simulink model "singlePhaseInverterOpenLoop"  (R2023a)
settings: Solver=VariableStepAuto  StartTime=0.0  StopTime=.2  FixedStep=1e-3  MaxStep=1e-5  RelTol=1e-3
libraries: spsIGBTDiodeLib x16, spsDCVoltageSourceLib x8, spsTHDLib x8, spsCurrentMeasurementLib x6, spsGroundLib x4, spsSeriesRLCBranchLib x4, spsVoltageMeasurementLib x4, spspowerguiLib x3, simulink x3, spsMeanLib x1, spsTriangleGeneratorLib x1
settings Model: Creator=User  LastModifiedBy=User
settings SolverCC: AlgebraicLoopSolver=TrustRegion
settings DebuggingCC: UnconnectedInputMsg=warning  UnconnectedOutputMsg=warning  UnconnectedLineMsg=warning
settings ModelReferenceCC: EnableRefExpFcnMdlSchedulingChecks=on
settings RTWCC: DLArmComputeVersion=19.05

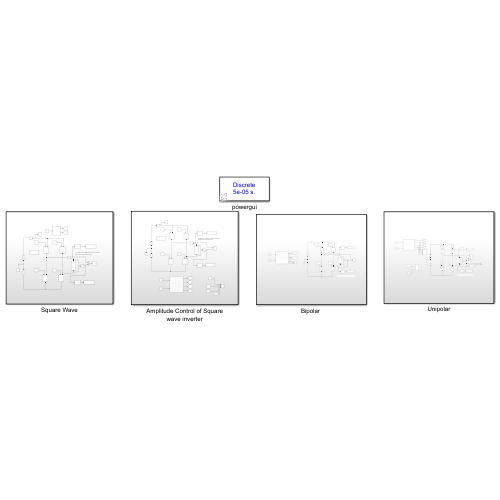
[thumbnail: Simulink's stored preview of the top-level diagram]
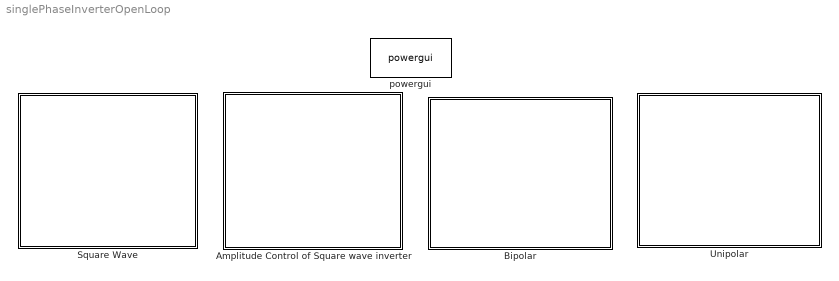
== system singlePhaseInverterOpenLoop ==
  Amplitude Control of Square wave inverter : Subsystem
  "Bipolar " : Subsystem
  Square Wave : Subsystem
  Unipolar : Subsystem
  powergui : spspowerguiLib/powergui  Priority=1  SimulationMode=Discrete  SampleTime=50e-6  frequency=60  Iterations=50  frequencyindice=0  Pbase=100e6  ErrMax=1e-4  UnitsV=kV  UnitsW=MW  buscounter=0  FunctionMessages=off  echomessages=off  EnableUseOfTLC=off  CurrentSourceSwitches=off  DisableSnubberDevices=on  DisableRonSwitches=on  DisableVfSwitches=on  DisplayEquations=off  AutomaticDiscreteSolvers=off  SolverType=Tustin/Backward Euler (TBE)  Interpol=off  ExternalGateDelay=off  methode=off  Ts=100  x0status=blocks  SPID=on  SwTol=0  HookPort=off  NonlinearTolerance=1e-4  nMaxIteration=100  ContinueOnMaxIteration=off  RestoreLinks=warning  ResistiveCurrentMeasurement=off  Frange=[0:2:500]  Ylog=off  Xlog=on  ShowGrid=off  save=off  variable=ZData  structure=0  ZoomFFT=off  StartTime=0.0  cycles=1  DisplayStyle=1  fundamental=60  FreqAxis=off  MaxFrequency=1000  frequencyindicesteady=1  RmsSteady=1  display=off

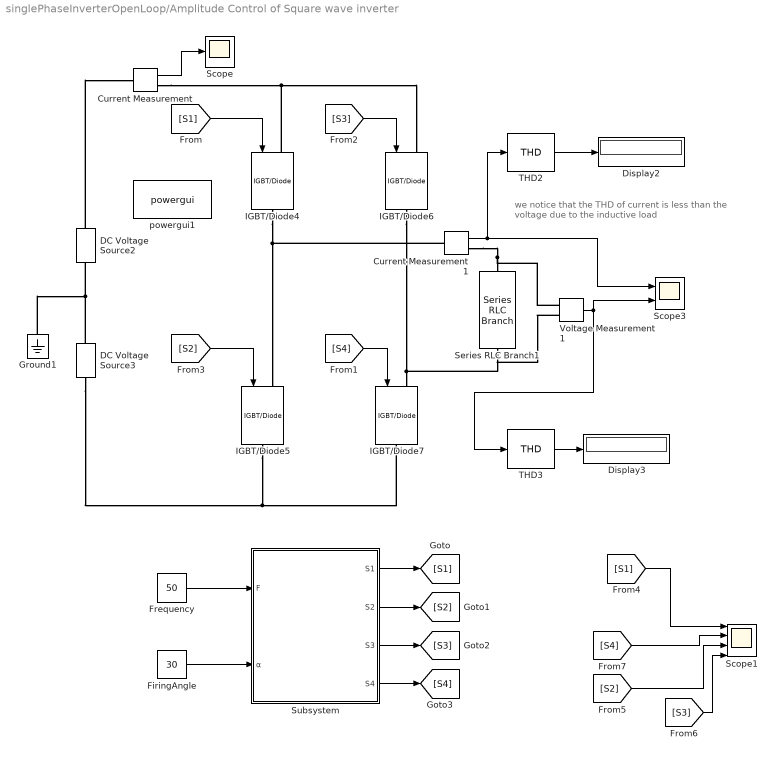
== system singlePhaseInverterOpenLoop/Amplitude Control of Square wave inverter ==
  note: we notice that the THD of current is less than the voltage due to the inductive load
  Current Measurement : spsCurrentMeasurementLib/Current Measurement  PhasorSimulation=off  OutputType=Complex  PSBequivalent=0
  Current Measurement1 : spsCurrentMeasurementLib/Current Measurement  PhasorSimulation=off  OutputType=Complex  PSBequivalent=0
  DC Voltage Source2 : spsDCVoltageSourceLib/DC Voltage Source  Amplitude=100  Measurements=None
  DC Voltage Source3 : spsDCVoltageSourceLib/DC Voltage Source  Amplitude=100  Measurements=None
  Display2 : Display
  Display3 : Display
  FiringAngle : Constant  Value=30
  Frequency : Constant  Value=50
  Ground1 : spsGroundLib/Ground  LConnTagsString=a
  IGBT/Diode{4..7} (4 alike) : spsIGBTDiodeLib/IGBT//Diode  Ron=1e-3  Rs=1e5  Cs=inf  Measurements=off
  Scope : Scope
  Scope1 : Scope  NumInputPorts=4
  Scope3 : Scope  NumInputPorts=2
  Series RLC Branch1 : spsSeriesRLCBranchLib/Series RLC Branch  LConnTagsString=__new0  RConnTagsString=__new0  BranchType=RL  Resistance=1  Inductance=1e-3  SetiL0=off  InitialCurrent=0  Capacitance=1e-6  Setx0=off  InitialVoltage=0  Measurements=None
  Subsystem : Subsystem
  THD2 : spsTHDLib/THD  Freq=60  Ts=0
  THD3 : spsTHDLib/THD  Freq=60  Ts=0
  Voltage Measurement1 : spsVoltageMeasurementLib/Voltage Measurement  PhasorSimulation=off  OutputType=Complex  PSBequivalent=0
  powergui1 : spspowerguiLib/powergui  Priority=1  SimulationMode=Continuous  SampleTime=50e-6  frequency=60  Iterations=50  frequencyindice=0  Pbase=100e6  ErrMax=1e-4  UnitsV=kV  UnitsW=MW  buscounter=0  FunctionMessages=off  echomessages=off  EnableUseOfTLC=off  CurrentSourceSwitches=off  DisableSnubberDevices=on  DisableRonSwitches=on  DisableVfSwitches=on  DisplayEquations=off  AutomaticDiscreteSolvers=off  SolverType=Tustin/Backward Euler (TBE)  Interpol=off  ExternalGateDelay=off  methode=off  Ts=100  x0status=blocks  SPID=on  SwTol=0  HookPort=off  NonlinearTolerance=1e-4  nMaxIteration=100  ContinueOnMaxIteration=off  RestoreLinks=warning  ResistiveCurrentMeasurement=off  Frange=[0:2:500]  Ylog=off  Xlog=on  ShowGrid=off  save=off  variable=ZData  structure=0  ZoomFFT=off  StartTime=0.0  cycles=1  DisplayStyle=1  fundamental=60  FreqAxis=off  MaxFrequency=1000  frequencyindicesteady=1  RmsSteady=1  display=off
  wires:
  Current Measurement/1 -> Scope/1
  [S1] -> IGBT/Diode4/1
  Voltage Measurement1/1 -> Scope3/2, THD3/1
  THD2/1 -> Display2/1
  [S2] -> IGBT/Diode5/1
  [S3] -> IGBT/Diode6/1
  THD3/1 -> Display3/1
  [S4] -> IGBT/Diode7/1
  Current Measurement1/1 -> Scope3/1, THD2/1
  Frequency/1 -> Subsystem/1(F)
  FiringAngle/1 -> Subsystem/2(α)
  Subsystem/1(S1) -> [S1]
  Subsystem/2(S2) -> [S2]
  Subsystem/3(S3) -> [S3]
  Subsystem/4(S4) -> [S4]
  [S1] -> Scope1/1
  [S2] -> Scope1/3
  [S3] -> Scope1/4
  [S4] -> Scope1/2
  connections:
  DC Voltage Source2/RConn1 -- Current Measurement/LConn1
  Voltage Measurement1/LConn1 -- Current Measurement1/RConn1 -- Series RLC Branch1/LConn1
  Ground1/LConn1 -- DC Voltage Source3/RConn1 -- DC Voltage Source2/LConn1
  IGBT/Diode6/RConn1 -- Series RLC Branch1/RConn1 -- Voltage Measurement1/LConn2 -- IGBT/Diode7/LConn1
  Current Measurement1/LConn1 -- IGBT/Diode4/RConn1 -- IGBT/Diode5/LConn1
  IGBT/Diode4/LConn1 -- Current Measurement/RConn1 -- IGBT/Diode6/LConn1
  DC Voltage Source3/LConn1 -- IGBT/Diode7/RConn1 -- IGBT/Diode5/RConn1

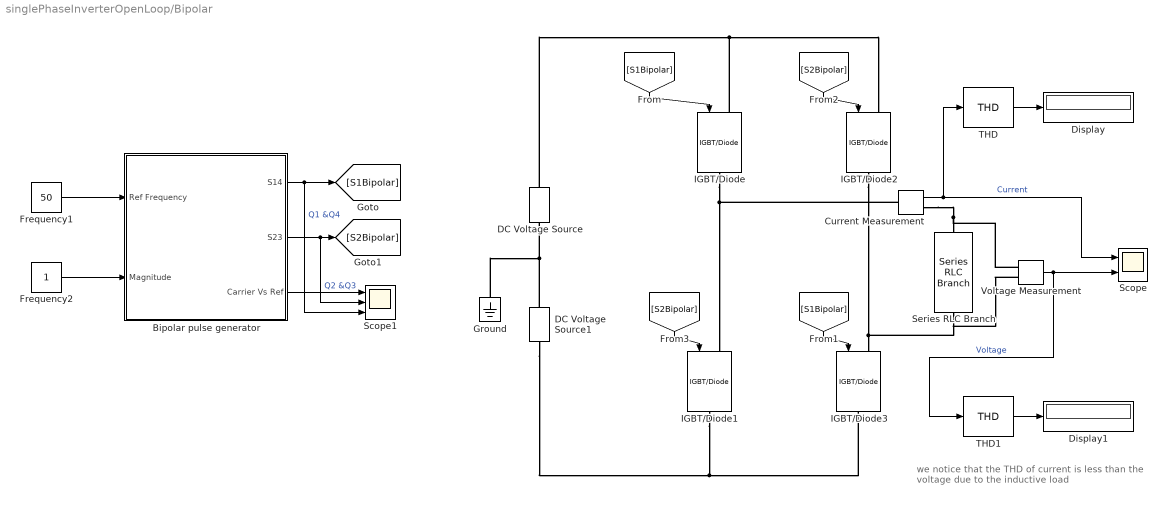
== system singlePhaseInverterOpenLoop/Bipolar  ==
  note: we notice that the THD of current is less than the voltage due to the inductive load
  Bipolar pulse generator : Subsystem
  Current Measurement : spsCurrentMeasurementLib/Current Measurement  PhasorSimulation=off  OutputType=Complex  PSBequivalent=0
  DC Voltage Source : spsDCVoltageSourceLib/DC Voltage Source  Amplitude=100  Measurements=None
  DC Voltage Source1 : spsDCVoltageSourceLib/DC Voltage Source  Amplitude=100  Measurements=None
  Display : Display
  Display1 : Display
  Frequency1 : Constant  Value=50
  Frequency2 : Constant
  Ground : spsGroundLib/Ground  LConnTagsString=a
  IGBT/Diode{,1..3} (4 alike) : spsIGBTDiodeLib/IGBT//Diode  Ron=1e-3  Rs=1e5  Cs=inf  Measurements=off
  Scope : Scope  NumInputPorts=2
  Scope1 : Scope  NumInputPorts=3
  Series RLC Branch : spsSeriesRLCBranchLib/Series RLC Branch  LConnTagsString=__new0  RConnTagsString=__new0  BranchType=RL  Resistance=1  Inductance=50e-3  SetiL0=off  InitialCurrent=0  Capacitance=1e-6  Setx0=off  InitialVoltage=0  Measurements=None
  THD : spsTHDLib/THD  Freq=60  Ts=0
  THD1 : spsTHDLib/THD  Freq=60  Ts=0
  Voltage Measurement : spsVoltageMeasurementLib/Voltage Measurement  PhasorSimulation=off  OutputType=Complex  PSBequivalent=0
  wires:
  THD/1 -> Display/1
  [S1Bipolar] -> IGBT/Diode3/1
  THD1/1 -> Display1/1
  [S1Bipolar] -> IGBT/Diode/1
  Current Measurement/1 -> Scope/1, THD/1  "Current"
  [S2Bipolar] -> IGBT/Diode2/1
  [S2Bipolar] -> IGBT/Diode1/1
  Voltage Measurement/1 -> Scope/2, THD1/1  "Voltage"
  Frequency1/1 -> Bipolar pulse generator/1(Ref Frequency)
  Bipolar pulse generator/1(S14) -> Scope1/3, [S1Bipolar]  "Q1 &Q4"
  Bipolar pulse generator/2(S23) -> Scope1/2, [S2Bipolar]  "Q2 &Q3"
  Frequency2/1 -> Bipolar pulse generator/2(Magnitude)
  Bipolar pulse generator/3(Carrier Vs Ref) -> Scope1/1
  connections:
  IGBT/Diode/LConn1 -- DC Voltage Source/RConn1 -- IGBT/Diode2/LConn1
  IGBT/Diode2/RConn1 -- Voltage Measurement/LConn2 -- Series RLC Branch/RConn1 -- IGBT/Diode3/LConn1
  IGBT/Diode/RConn1 -- Current Measurement/LConn1 -- IGBT/Diode1/LConn1
  IGBT/Diode1/RConn1 -- IGBT/Diode3/RConn1 -- DC Voltage Source1/LConn1
  DC Voltage Source1/RConn1 -- Ground/LConn1 -- DC Voltage Source/LConn1
  Current Measurement/RConn1 -- Voltage Measurement/LConn1 -- Series RLC Branch/LConn1

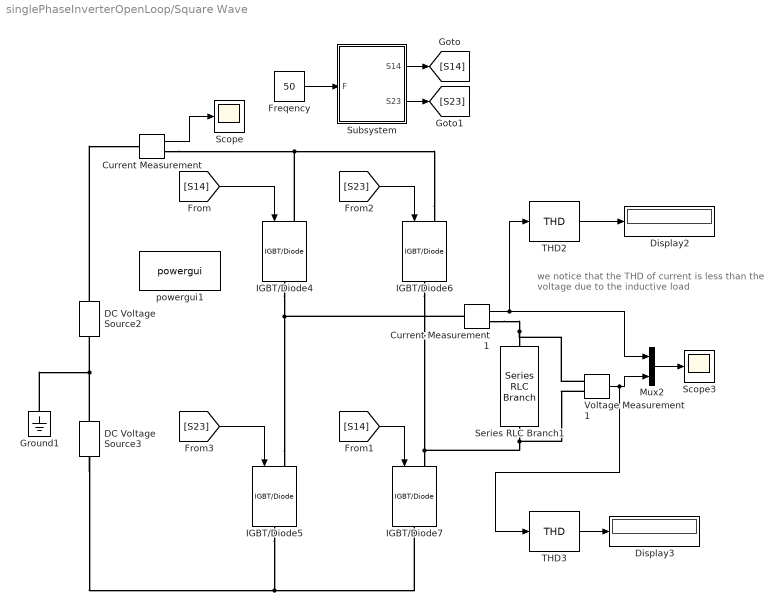
== system singlePhaseInverterOpenLoop/Square Wave ==
  note: we notice that the THD of current is less than the voltage due to the inductive load
  Current Measurement : spsCurrentMeasurementLib/Current Measurement  PhasorSimulation=off  OutputType=Complex  PSBequivalent=0
  Current Measurement1 : spsCurrentMeasurementLib/Current Measurement  PhasorSimulation=off  OutputType=Complex  PSBequivalent=0
  DC Voltage Source2 : spsDCVoltageSourceLib/DC Voltage Source  Amplitude=100  Measurements=None
  DC Voltage Source3 : spsDCVoltageSourceLib/DC Voltage Source  Amplitude=100  Measurements=None
  Display2 : Display
  Display3 : Display
  Freqency : Constant  Value=50
  Ground1 : spsGroundLib/Ground  LConnTagsString=a
  IGBT/Diode{4..7} (4 alike) : spsIGBTDiodeLib/IGBT//Diode  Ron=1e-3  Rs=1e5  Cs=inf  Measurements=off
  Mux2 : Mux  Inputs=2
  Scope : Scope
  Scope3 : Scope
  Series RLC Branch1 : spsSeriesRLCBranchLib/Series RLC Branch  LConnTagsString=__new0  RConnTagsString=__new0  BranchType=RL  Resistance=1  Inductance=50e-3  SetiL0=off  InitialCurrent=0  Capacitance=1e-6  Setx0=off  InitialVoltage=0  Measurements=None
  Subsystem : Subsystem
  THD2 : spsTHDLib/THD  Freq=60  Ts=0
  THD3 : spsTHDLib/THD  Freq=60  Ts=0
  Voltage Measurement1 : spsVoltageMeasurementLib/Voltage Measurement  PhasorSimulation=off  OutputType=Complex  PSBequivalent=0
  powergui1 : spspowerguiLib/powergui  Priority=1  SimulationMode=Continuous  SampleTime=50e-6  frequency=60  Iterations=50  frequencyindice=0  Pbase=100e6  ErrMax=1e-4  UnitsV=kV  UnitsW=MW  buscounter=0  FunctionMessages=off  echomessages=off  EnableUseOfTLC=off  CurrentSourceSwitches=off  DisableSnubberDevices=on  DisableRonSwitches=on  DisableVfSwitches=on  DisplayEquations=off  AutomaticDiscreteSolvers=off  SolverType=Tustin/Backward Euler (TBE)  Interpol=off  ExternalGateDelay=off  methode=off  Ts=100  x0status=blocks  SPID=on  SwTol=0  HookPort=off  NonlinearTolerance=1e-4  nMaxIteration=100  ContinueOnMaxIteration=off  RestoreLinks=warning  ResistiveCurrentMeasurement=off  Frange=[0:2:500]  Ylog=off  Xlog=on  ShowGrid=off  save=off  variable=ZData  structure=0  ZoomFFT=off  StartTime=0.0  cycles=1  DisplayStyle=1  fundamental=60  FreqAxis=off  MaxFrequency=1000  frequencyindicesteady=1  RmsSteady=1  display=off
  wires:
  Current Measurement1/1 -> Mux2/1, THD2/1
  Mux2/1 -> Scope3/1
  [S14] -> IGBT/Diode7/1
  THD3/1 -> Display3/1
  [S23] -> IGBT/Diode6/1
  [S23] -> IGBT/Diode5/1
  THD2/1 -> Display2/1
  Voltage Measurement1/1 -> THD3/1, Mux2/2
  [S14] -> IGBT/Diode4/1
  Freqency/1 -> Subsystem/1(F)
  Subsystem/2(S23) -> [S23]
  Subsystem/1(S14) -> [S14]
  Current Measurement/1 -> Scope/1
  connections:
  IGBT/Diode5/RConn1 -- IGBT/Diode7/RConn1 -- DC Voltage Source3/LConn1
  IGBT/Diode6/LConn1 -- Current Measurement/RConn1 -- IGBT/Diode4/LConn1
  IGBT/Diode5/LConn1 -- IGBT/Diode4/RConn1 -- Current Measurement1/LConn1
  IGBT/Diode7/LConn1 -- Voltage Measurement1/LConn2 -- Series RLC Branch1/RConn1 -- IGBT/Diode6/RConn1
  DC Voltage Source2/LConn1 -- DC Voltage Source3/RConn1 -- Ground1/LConn1
  Series RLC Branch1/LConn1 -- Current Measurement1/RConn1 -- Voltage Measurement1/LConn1
  DC Voltage Source2/RConn1 -- Current Measurement/LConn1

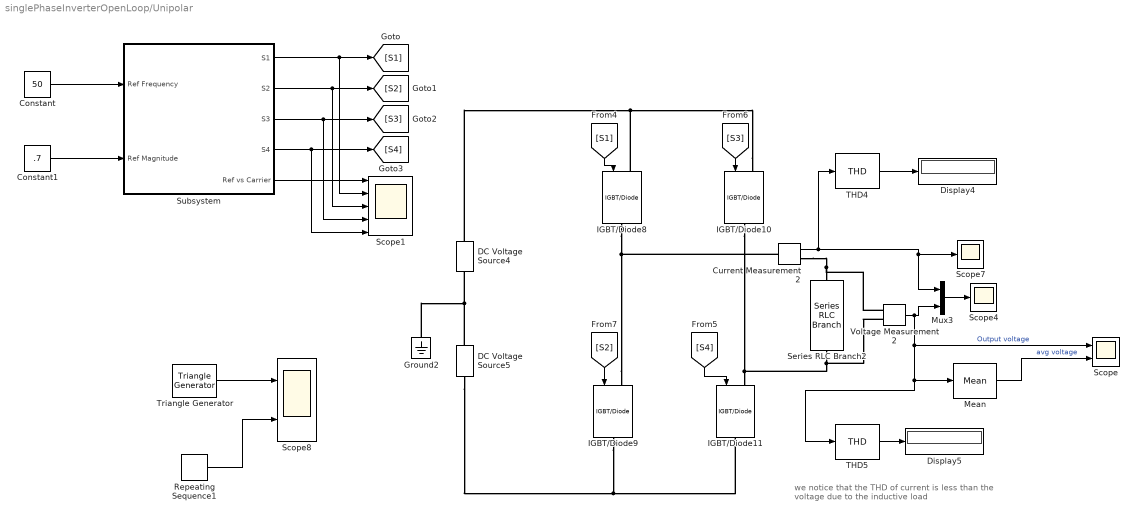
== system singlePhaseInverterOpenLoop/Unipolar ==
  note: we notice that the THD of current is less than the voltage due to the inductive load
  Constant : Constant  Value=50
  Constant1 : Constant  Value=.7
  Current Measurement2 : spsCurrentMeasurementLib/Current Measurement  PhasorSimulation=off  OutputType=Complex  PSBequivalent=0
  DC Voltage Source4 : spsDCVoltageSourceLib/DC Voltage Source  Amplitude=100  Measurements=None
  DC Voltage Source5 : spsDCVoltageSourceLib/DC Voltage Source  Amplitude=100  Measurements=None
  Display4 : Display
  Display5 : Display
  Ground2 : spsGroundLib/Ground  LConnTagsString=a
  IGBT/Diode{8..11} (4 alike) : spsIGBTDiodeLib/IGBT//Diode  Ron=1e-3  Rs=1e5  Cs=inf  Measurements=off
  Mean : spsMeanLib/Mean  Freq=60  Vinit=0  Ts=0
  Mux3 : Mux  Inputs=2
  "Repeating Sequence1  " : simulink/Sources/Repeating Sequence  rep_seq_t=[0 1 2 3 4]*[1/400]  rep_seq_y=[0 1 0 -1 0]
  Scope : Scope  NumInputPorts=2
  Scope1 : Scope  NumInputPorts=5
  Scope4 : Scope
  Scope7 : Scope
  Scope8 : Scope  NumInputPorts=2
  Series RLC Branch2 : spsSeriesRLCBranchLib/Series RLC Branch  LConnTagsString=__new0  RConnTagsString=__new0  BranchType=RL  Resistance=1  Inductance=50e-3  SetiL0=off  InitialCurrent=0  Capacitance=1e-6  Setx0=off  InitialVoltage=0  Measurements=None
  Subsystem : Subsystem
  THD4 : spsTHDLib/THD  Freq=60  Ts=0
  THD5 : spsTHDLib/THD  Freq=60  Ts=0
  "Triangle Generator " : spsTriangleGeneratorLib/Triangle Generator  Freq=1e2  Phase=0  Ts=0
  Voltage Measurement2 : spsVoltageMeasurementLib/Voltage Measurement  PhasorSimulation=off  OutputType=Complex  PSBequivalent=0
  wires:
  Current Measurement2/1 -> Mux3/1, Scope7/1, THD4/1
  [S1] -> IGBT/Diode8/1
  Mux3/1 -> Scope4/1
  Voltage Measurement2/1 -> Scope/1, Mean/1, THD5/1, Mux3/2  "Output voltage"
  [S3] -> IGBT/Diode10/1
  [S2] -> IGBT/Diode9/1
  [S4] -> IGBT/Diode11/1
  "Triangle Generator "/1 -> Scope8/1
  THD4/1 -> Display4/1
  "Repeating Sequence1  "/1 -> Scope8/2
  THD5/1 -> Display5/1
  Subsystem/1(S1) -> Scope1/2, [S1]
  Subsystem/2(S2) -> Scope1/3, [S2]
  Subsystem/3(S3) -> Scope1/4, [S3]
  Subsystem/4(S4) -> Scope1/5, [S4]
  Constant/1 -> Subsystem/1(Ref Frequency)
  Subsystem/5(Ref vs Carrier) -> Scope1/1
  Constant1/1 -> Subsystem/2(Ref Magnitude)
  Mean/1 -> Scope/2  "avg voltage"
  connections:
  IGBT/Diode9/RConn1 -- DC Voltage Source5/LConn1 -- IGBT/Diode11/RConn1
  DC Voltage Source4/LConn1 -- DC Voltage Source5/RConn1 -- Ground2/LConn1
  IGBT/Diode11/LConn1 -- Voltage Measurement2/LConn2 -- Series RLC Branch2/RConn1 -- IGBT/Diode10/RConn1
  IGBT/Diode9/LConn1 -- IGBT/Diode8/RConn1 -- Current Measurement2/LConn1
  Series RLC Branch2/LConn1 -- Current Measurement2/RConn1 -- Voltage Measurement2/LConn1
  IGBT/Diode10/LConn1 -- DC Voltage Source4/RConn1 -- IGBT/Diode8/LConn1

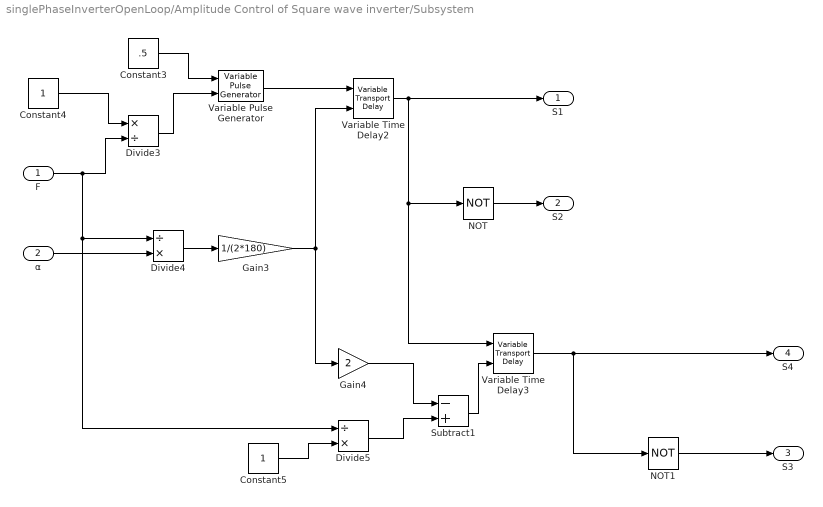
== system singlePhaseInverterOpenLoop/Amplitude Control of Square wave inverter/Subsystem ==
  F : Inport
  α : Inport  Port=2
  Constant3 : Constant  Value=.5
  Constant4 : Constant
  Constant5 : Constant
  Divide3 : Product  Inputs=*/
  Divide4 : Product  Inputs=/*
  Divide5 : Product  Inputs=/*
  Gain3 : Gain  Gain=1/(2*180)
  Gain4 : Gain  Gain=2
  NOT : Logic  Operator=NOT  IconShape=distinctive  AllPortsSameDT=off  OutDataTypeStr=boolean
  NOT1 : Logic  Operator=NOT  IconShape=distinctive  AllPortsSameDT=off  OutDataTypeStr=boolean
  Subtract1 : Sum  Inputs=-+
  Variable Time Delay2 : VariableTransportDelay  MaximumDelay=10  MaximumPoints=3072
  Variable Time Delay3 : VariableTransportDelay  MaximumDelay=10  MaximumPoints=3072
  Variable Pulse Generator : VariablePulseGenerator  SampleTime=0.1
  S1 : Outport
  S2 : Outport  Port=2
  S3 : Outport  Port=3
  S4 : Outport  Port=4
  wires:
  F/1 -> Divide5/1, Divide4/1, Divide3/2
  Constant3/1 -> Variable Pulse Generator/1
  Divide5/1 -> Subtract1/2
  Variable Pulse Generator/1 -> Variable Time Delay2/1
  α/1 -> Divide4/2
  Constant5/1 -> Divide5/2
  Constant4/1 -> Divide3/1
  Variable Time Delay2/1 -> Variable Time Delay3/1, NOT/1, S1/1
  Divide3/1 -> Variable Pulse Generator/2
  Divide4/1 -> Gain3/1
  Subtract1/1 -> Variable Time Delay3/2
  Gain4/1 -> Subtract1/1
  Gain3/1 -> Gain4/1, Variable Time Delay2/2
  NOT/1 -> S2/1
  Variable Time Delay3/1 -> NOT1/1, S4/1
  NOT1/1 -> S3/1

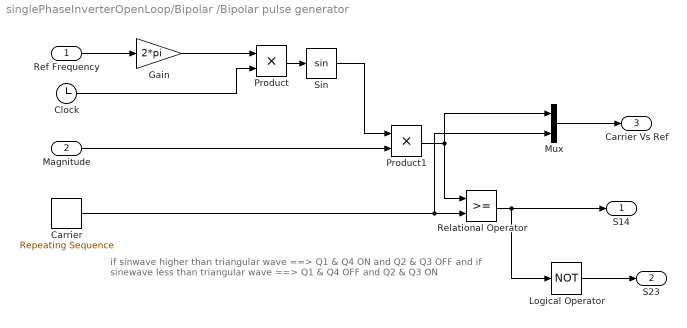
== system singlePhaseInverterOpenLoop/Bipolar /Bipolar pulse generator ==
  note: if sinwave higher than triangular wave ==> Q1 & Q4 ON and Q2 & Q3 OFF
      | and if sinewave less than triangular wave ==> Q1 & Q4 OFF and Q2 & Q3 ON
  Ref Frequency : Inport
  Magnitude : Inport  Port=2
  Carrier : simulink/Sources/Repeating Sequence  rep_seq_t=[0 1 2 3 4]*[1/500]  rep_seq_y=[0 1 0 -1 0]
  Clock : Clock
  Gain : Gain  Gain=2*pi
  Logical Operator : Logic  Operator=NOT  AllPortsSameDT=off  OutDataTypeStr=boolean
  Mux : Mux  Inputs=2
  Product : Product
  Product1 : Product
  Relational Operator : RelationalOperator  OutDataTypeStr=boolean  RndMeth=Simplest  InputSameDT=off
  Sin : Trigonometry
  S14 : Outport
  S23 : Outport  Port=2
  Carrier Vs Ref : Outport  Port=3
  wires:
  Sin/1 -> Product1/1
  Clock/1 -> Product/2
  Gain/1 -> Product/1
  Product/1 -> Sin/1
  Logical Operator/1 -> S23/1
  Relational Operator/1 -> S14/1, Logical Operator/1
  Carrier/1 -> Mux/2, Relational Operator/2
  Ref Frequency/1 -> Gain/1
  Product1/1 -> Relational Operator/1, Mux/1
  Magnitude/1 -> Product1/2
  Mux/1 -> Carrier Vs Ref/1

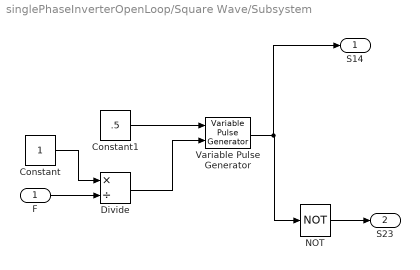
== system singlePhaseInverterOpenLoop/Square Wave/Subsystem ==
  F : Inport
  Constant : Constant
  Constant1 : Constant  Value=.5
  Divide : Product  Inputs=*/
  NOT : Logic  Operator=NOT  IconShape=distinctive  AllPortsSameDT=off  OutDataTypeStr=boolean
  Variable Pulse Generator : VariablePulseGenerator  SampleTime=0.1
  S14 : Outport
  S23 : Outport  Port=2
  wires:
  Divide/1 -> Variable Pulse Generator/2
  Variable Pulse Generator/1 -> S14/1, NOT/1
  Constant1/1 -> Variable Pulse Generator/1
  Constant/1 -> Divide/1
  NOT/1 -> S23/1
  F/1 -> Divide/2

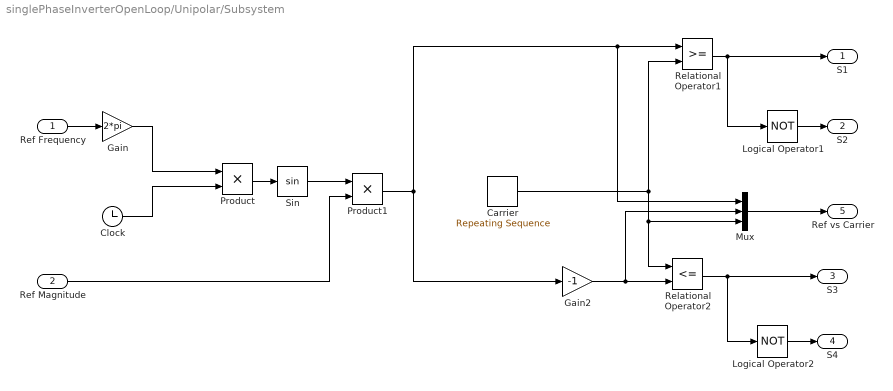
== system singlePhaseInverterOpenLoop/Unipolar/Subsystem ==
  Ref Frequency : Inport
  Ref Magnitude : Inport  Port=2
  Carrier : simulink/Sources/Repeating Sequence  rep_seq_t=[0 1 2 3 4]*[1/5000]  rep_seq_y=[0 1 0 -1 0]
  Clock : Clock
  Gain : Gain  Gain=2*pi
  Gain2 : Gain  Gain=-1
  Logical Operator1 : Logic  Operator=NOT  AllPortsSameDT=off  OutDataTypeStr=boolean
  Logical Operator2 : Logic  Operator=NOT  AllPortsSameDT=off  OutDataTypeStr=boolean
  Mux : Mux  Inputs=3
  Product : Product
  Product1 : Product
  Relational Operator1 : RelationalOperator  OutDataTypeStr=boolean  RndMeth=Simplest  InputSameDT=off
  Relational Operator2 : RelationalOperator  Operator=<=  OutDataTypeStr=boolean  RndMeth=Simplest  InputSameDT=off
  Sin : Trigonometry
  S1 : Outport
  S2 : Outport  Port=2
  S3 : Outport  Port=3
  S4 : Outport  Port=4
  Ref vs Carrier : Outport  Port=5
  wires:
  Carrier/1 -> Mux/3, Relational Operator2/1, Relational Operator1/2
  Logical Operator1/1 -> S2/1
  Relational Operator2/1 -> S3/1, Logical Operator2/1
  Relational Operator1/1 -> S1/1, Logical Operator1/1
  Logical Operator2/1 -> S4/1
  Clock/1 -> Product/2
  Ref Frequency/1 -> Gain/1
  Gain/1 -> Product/1
  Product/1 -> Sin/1
  Product1/1 -> Mux/1, Relational Operator1/1, Gain2/1
  Gain2/1 -> Mux/2, Relational Operator2/2
  Sin/1 -> Product1/1
  Ref Magnitude/1 -> Product1/2
  Mux/1 -> Ref vs Carrier/1
